simulink model "rotated_stars"  (R2023b)
settings: Solver=VariableStepAuto  StartTime=0.0  StopTime=10.0  RelTol=1e-3
undefined symbols (not defined in the file): N, stars
libraries: sensors_subsystems x1
settings Model: Creator=brent  LastModifiedBy=brent

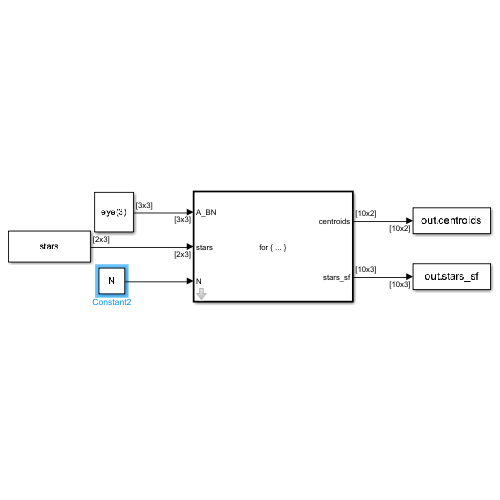
[thumbnail: Simulink's stored preview of the top-level diagram]
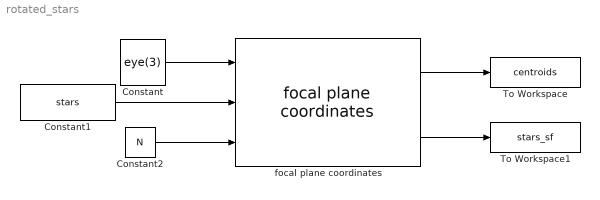
== system rotated_stars ==
  Constant : Constant  Value=eye(3)
  Constant1 : Constant  Value=stars
  Constant2 : Constant  Value=N
  To Workspace : ToWorkspace  VariableName=centroids  SampleTime=-1
      settings: Save2DSignal=2-D array (concatenate along first dimension)
  To Workspace1 : ToWorkspace  VariableName=stars_sf  SampleTime=-1
      settings: Save2DSignal=2-D array (concatenate along first dimension)
  focal plane coordinates : sensors_subsystems/focal plane coordinates  starTracker=starTracker
      settings: SourceProductName=Sensors library
  wires:
  Constant/1 -> focal plane coordinates/1
  Constant1/1 -> focal plane coordinates/2
  focal plane coordinates/1 -> To Workspace/1
  focal plane coordinates/2 -> To Workspace1/1
  Constant2/1 -> focal plane coordinates/3
